simulink model "pmc_vlpr_s32k14x"  (Simulink 9.0)
settings: Solver=FixedStepDiscrete  StartTime=0.0  StopTime=10.0  FixedStep=0.001  RelTol=1e-3
InitFcn:
  | mbd_s32k_consistency_checks(bdroot(gcs));
undefined symbols (not defined in the file): LQFP
libraries: mbd_s32k1xx_ec_toolbox x14, simulink x1
Description:
  | This model demonstrates the "VLPR" functionality by setting the
  | processor to run in the Very low power run (VLPR) mode. When the SW3 button is
  | pressed, the processor runs into the VLPR mode. To exit the VLPR mode to RUN mode
  | SW2 button must be pressed.
  | 
  | Attention: The VLPR mode  disables most of the clocks. Using LPIT timer as interrupt
  | for the step function causes to halt processor when the VLPR mode is switched on. This
  | model uses VLPR timer (clocked by SIRC which is on in VLPR mode) as step function
  | trigger so the Step Tick Timer must be suppressed.
  | 
  | Validation: When the processor boots up, the RGB led lights up green and the processor
  | runs in the RUN mode. The RGB will toggle blue every half a second. When the SW3 is
  | pressed the processor enters the VLPR mode and the RGB turns red. The Blue light will
  | continue to toggle. When the SW2 is pressed the processor toggles the RGB led green and
  | the processor will run in RUN mode.
  | 
  | Optional: In order to measure the current consumption of the processor you can desolder
  | the R117 resistor (on the S32K144EVB board) and attach an ammeter on the J15 jumper.
  | 
  | Warning: Do NOT program the board while the uC is running in the low poer mode!
settings Model: Creator=NXP MBDT Team  LastModifiedBy=nxf35172
settings DataIOCC: ExternalInput=off  InitialState=off  SaveFormat=Dataset  SaveOutput=off  SignalLogging=off  SaveTime=off
settings OptimizationCC: DefaultParameterBehavior=Inlined  LifeSpan=1
settings DebuggingCC: UnderspecifiedInitializationDetection=Simplified  MergeDetectMultiDrivingBlocksExec=error  InheritedTsInSrcMsg=none  SingleTaskRateTransMsg=error  ParameterTunabilityLossMsg=error  UnconnectedInputMsg=error  UnconnectedOutputMsg=error  UnconnectedLineMsg=error  UnknownTsInhSupMsg=error  SFUnexpectedBacktrackingDiag=error  SFNoUnconditionalDefaultTransitionDiag=error
settings HardwareCC: ProdLargestAtomicInteger=Long  ProdLargestAtomicFloat=Double  ProdIntDivRoundTo=Zero  ProdEndianess=LittleEndian  ProdHWDeviceType=ARM Compatible->ARM Cortex
settings ModelReferenceCC: PropagateSignalLabelsOutOfModel=on
settings SFSimCC: SimBuildMode=sf_nonincremental_build  MATLABDynamicMemAlloc=off
settings RTWCC: SystemTargetFile=mbd_s32k.tlc  MakeCommand=mbd_s32k_make_rtw COPY_MDLREF_INCLUDES=0  TemplateMakefile=mbd_s32k.tmf  Description=Model Based Design Toolbox S32K14x Code Generation Target  GenerateReport=on  RetainRTWFile=on  IncludeHyperlinkInReport=on  LaunchReport=on  GenerateTraceInfo=on  GenerateTraceReport=on  GenerateTraceReportSl=on  GenerateTraceReportSf=on  GenerateTraceReportEml=on
settings CodeAppCC: ForceParamTrailComments=on  IgnoreCustomStorageClasses=off  OperatorAnnotations=on  SimulinkDataObjDesc=on  SFDataObjDesc=on  MATLABFcnDesc=on  InsertBlockDesc=on  MATLABSourceComments=on
settings STFCustomTargetCC: CombineOutputUpdateFcns=on  ERTCustomFileBanners=on  SupportContinuousTime=off  SupportNonInlinedSFcns=off  RemoveResetFunc=on  MATLABClassNameForMDSCustomization=Simulink.SoftwareTarget.ERTCustomization  GRTInterface=off  SystemTargetFile=mbd_s32k14.tlc
settings ERTTargetCC: MultiwordLength=2048  ParMdlRefBuildCompliant=off  CompOptLevelCompliant=off  ConcurrentExecutionCompliant=off  ModelStepFunctionPrototypeControlCompliant=off  CPPClassGenCompliant=off  UseToolchainInfoCompliant=off  InlinedParameterPlacement=NonHierarchical  ERTCustomFileTemplate=example_file_process.tlc  ConvertIfToSwitch=off  SuppressUnreachableDefaultCases=off
settings ConfigComp: CovMetricSettings=dwe  CovHtmlReporting=off  CovSaveCumulativeToWorkspaceVar=off  CovSaveSingleToWorkspaceVar=off  CovExternalEMLEnable=on

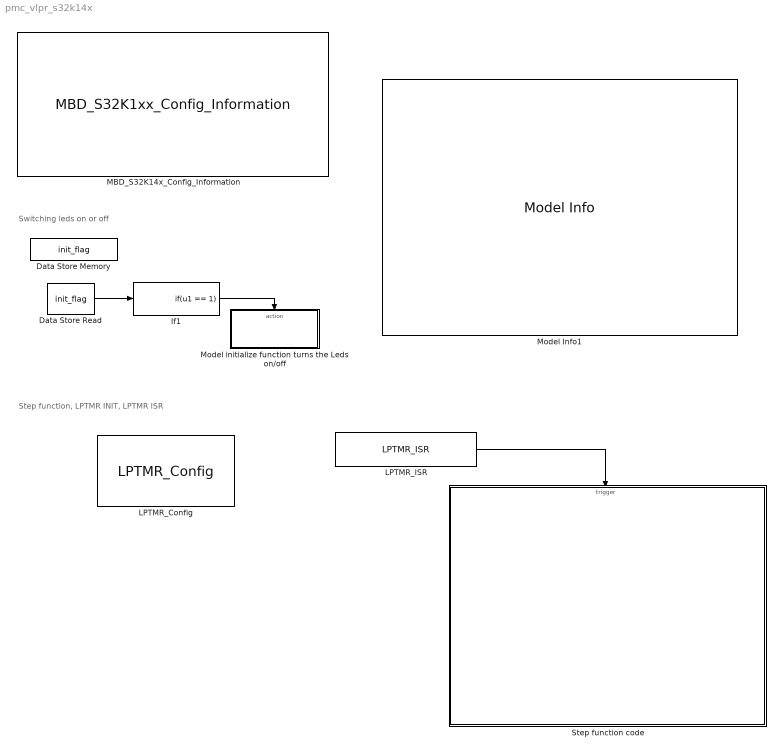
== system pmc_vlpr_s32k14x ==
  note: Switching leds on or off
  note: Step function, LPTMR INIT, LPTMR ISR
  Data Store Memory : DataStoreMemory  DataStoreName=init_flag  ReadBeforeWriteMsg=warning  WriteAfterWriteMsg=warning  WriteAfterReadMsg=warning  InitialValue=1  ShowAdditionalParam=off  OutDataTypeStr=boolean
  Data Store Read : DataStoreRead  DataStoreName=init_flag
  If1 : If  IfExpression=u1 == 1  ShowElse=off
  LPTMR_Config : mbd_s32k1xx_ec_toolbox/Core and System Blocks/LPTMR Blocks/LPTMR_Config  work_mode=Time Counter mode  compare_value=1000  compare_value_units=Microseconds  pin_select=Count pulses from pin alternative 1  pin_polarity=Count pulse on rising edge  pin_trgmux_source=Trigger function is disabled  pin_gpio=PTE11: [LPTMR0_ALT1 | Low Power Timer Input Channel]  show_adv_opts=on  input_clock=SIRC DIV2 clock  prescaler=Timer mode: prescaler 2, Glitch filter mode: invalid  bypass_prescaler=off  free_run=off  start_counter=on  enable_isr=on
  LPTMR_ISR : mbd_s32k1xx_ec_toolbox/Core and System Blocks/LPTMR Blocks/LPTMR_ISR
  MBD_S32K14x_Config_Information : mbd_s32k1xx_ec_toolbox/MBD_S32K1xx_Config_Information  mbdt_ver=0  disp_str=|  config_params=[]  mcu_target_name=S32K144  mcu_target_package=100-LQFP  mcu_target_sram_size=64KB  mcu_system_clock_freq=80  mcu_xtal_freq=External 8  mcu_steptick_timer=LPIT Channel 0  mcu_steptick_prio=15  ds_import_enable=on  target_compiler=GCC  target_memory=FLASH  gcc_target_compile_opts=-mcpu=cortex-m4 -mthumb -mfloat-abi=hard -mfpu=fpv4-sp-d16 -O1 -g -gstrict-dwarf  gcc_target_assemble_opts=-mcpu=cortex-m4 -mthumb -mfloat-abi=hard -mfpu=fpv4-sp-d16 -g  gcc_target_link_opts=-mcpu=cortex-m4 -mthumb -mfloat-abi=hard -mfpu=fpv4-sp-d16  gcc_target_default_lcf=on  gcc_target_user_lcf=S32K144_64_flash.ld  ghs_target_compile_opts=-cpu=cortexm4f -thumb -DARM_MATH_CM4 -fpu=vfpv4_d16 -fsingle -Ogeneral -Wundef -Wimplicit-int -Wshadow -Wtrigraphs --no_commons --gnu_asm -gnu99 -gdwarf-2 -G  ghs_target_assemble_opts=-cpu=cortexm4f -fpu=vfpv4_d16  ghs_target_link_opts=-cpu=cortexm4f -thumb -fpu=vfpv4_d16  ghs_target_default_lcf=on  ghs_target_user_lcf=S32K144_64_flash.ld  iar_target_compile_opts=--cpu=Cortex-M4F --thumb --fpu=VFPv4_sp -Ol -e --debug --dlib_config normal  iar_target_assemble_opts=--cpu Cortex-M4F --thumb --fpu VFPv4_sp  iar_target_link_opts=--no_exceptions --vfe --inline  iar_target_default_lcf=on  iar_target_user_lcf=S32K144_64_flash.icf  pil_download_enable=off  rbl_download_enable=on  rbl_start_delay=5000000  rbl_download_interface=OpenSDA  rbl_restart_request=off  rbl_com_port=Custom  rbl_com_port_custom=COM1  pil_download_rate=57600  pil_opensda_drive=Custom  pil_opensda_drive_custom=D  pil_uart_instance=0  pil_uart_rx=PTA2: [LPUART0_RX | Receive]  pil_uart_tx=PTA3: [LPUART0_TX | Transmit]  FTM_PWM_PcrCheckEnDis=on  FTM_Input_Edge_Inputs_PcrCheckEnDis=on  FTM_Dual_Edge_Inputs_PcrCheckEnDis=on  FTM_Quadrature_Inputs_PcrCheckEnDis=on  FTM_Hall_Sensor_Inputs_PcrCheckEnDis=on  LPTMR_PcrCheckEnDis=on  PIT_PcrCheckEnDis=on  RTC_PcrCheckEnDis=on  FlexCAN_PcrCheckEnDis=on  LIN_PcrCheckEnDis=on  FlexIO_PcrCheckEnDis=on  LPI2C_PcrCheckEnDis=on  LPSPI_PcrCheckEnDis=on  LPUART_PcrCheckEnDis=on  CMP_PcrCheckEnDis=on  GPIO_OutputPcrCheckEnDis=on  GPIO_InputPcrCheckEnDis=on  SBC_PcrCheckEnDis=on  AMMCLIB_PcrCheckEnDis=on  FM_PcrCheckEnDis=on  Profile_PcrCheckEnDis=on  ConfigParams_PcrCheckEnDis=on  ModelRef_PcrCheckEnDis=on  PDB0_PcrCheckEnDis=on  CSEc_PcrCheckEnDis=on  eDMA_PcrCheckEnDis=on  ADC_PcrCheckEnDis=on  WDOG_PcrCheckEnDis=on
      | Target : S32K144-64KB_SRAM
      | Package : 100-pin
      | System clock : 80 MHz
      | XTAL clock : External 8 MHz
      | Compiler : GCC
      | Target Type : FLASH
      | Download Code after build : (OpenSDA: D)
      | Step Tick Interrupt Priority : 10
  Model Info1 : simulink/Model-Wide Utilities/Model Info  Frame=off  DisplayStringWithTags=|  HorizontalTextAlignment=Left  LeftAlignmentValue=0.02
      | Model Name: %<ModelName>
      | 
      | Description: %<Description>
  Model initialize function turns the Leds on/off : Subsystem  TreatAsAtomicUnit=on
  Step function code : Subsystem
  wires:
  LPTMR_ISR/1 -> Step function code/Trigger
  Data Store Read/1 -> If1/1
  If1/1 -> Model initialize function turns the Leds on/off/Action

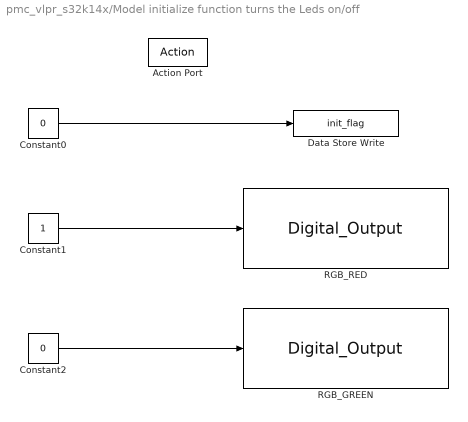
== system pmc_vlpr_s32k14x/Model initialize function turns the Leds on/off ==
  Action Port : ActionPort
  Constant0 : Constant  Value=0  OutDataTypeStr=boolean
  Constant1 : Constant  OutDataTypeStr=boolean
  Constant2 : Constant  Value=0  OutDataTypeStr=boolean
  Data Store Write : DataStoreWrite  DataStoreName=init_flag
  RGB_GREEN : mbd_s32k1xx_ec_toolbox/GPIO Blocks/Digital_Output  gpio_pin=PTD16: [PTD16 | Port D I/O]  init_val=Low  drive_strength=Low
  "RGB_RED " : mbd_s32k1xx_ec_toolbox/GPIO Blocks/Digital_Output  gpio_pin=PTD15: [PTD15 | Port D I/O]  init_val=Low  drive_strength=Low
  wires:
  Constant1/1 -> "RGB_RED "/1
  Constant0/1 -> Data Store Write/1
  Constant2/1 -> RGB_GREEN/1

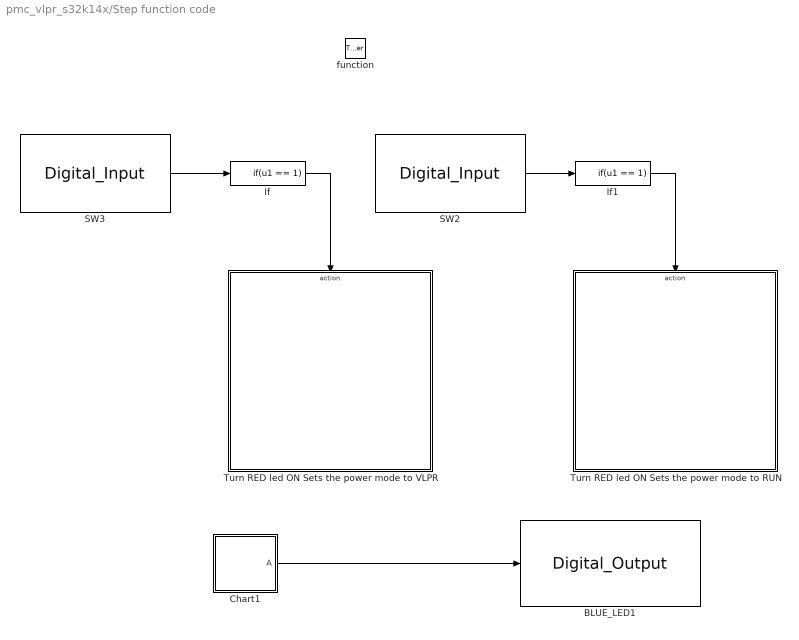
== system pmc_vlpr_s32k14x/Step function code ==
  function : TriggerPort  TriggerType=function-call  VariantControl=Variant
  BLUE_LED1 : mbd_s32k1xx_ec_toolbox/GPIO Blocks/Digital_Output  gpio_pin=PTD0: [PTD0 | Port D I/O]  init_val=Low  drive_strength=Low
  Chart1 : Stateflow chart  TreatAsAtomicUnit=on
  If : If  IfExpression=u1 == 1  ShowElse=off
  If1 : If  IfExpression=u1 == 1  ShowElse=off
  SW2 : mbd_s32k1xx_ec_toolbox/GPIO Blocks/Digital_Input  gpio_pin=PTC12: [PTC12 | Port C I/O]  pull_resistor=None  passive_filter=on
  SW3 : mbd_s32k1xx_ec_toolbox/GPIO Blocks/Digital_Input  gpio_pin=PTC13: [PTC13 | Port C I/O]  pull_resistor=None  passive_filter=on
  Turn RED led ON Sets the power mode to RUN : Subsystem  TreatAsAtomicUnit=on
  Turn RED led ON Sets the power mode to VLPR : Subsystem  TreatAsAtomicUnit=on
  wires:
  Chart1/1(" A") -> BLUE_LED1/1
  SW3/1 -> If/1
  If/1 -> Turn RED led ON Sets the power mode to VLPR/Action
  SW2/1 -> If1/1
  If1/1 -> Turn RED led ON Sets the power mode to RUN/Action

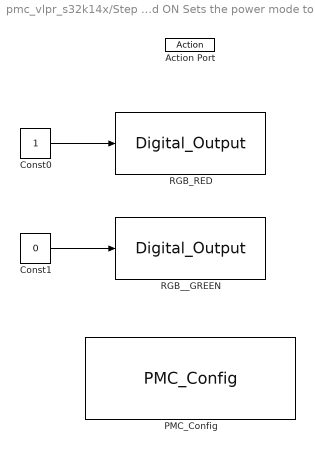
== system pmc_vlpr_s32k14x/Step function code/Turn RED led ON Sets the power mode to RUN ==
  Action Port : ActionPort
  Const0 : Constant  OutDataTypeStr=boolean
  Const1 : Constant  Value=0  OutDataTypeStr=boolean
  PMC_Config : mbd_s32k1xx_ec_toolbox/Core and System Blocks/PMC Blocks/PMC_Config  power_mode=Normal Operating (RUN)  sleep_on_exit=off  callback_before=off  callback_after=off  callback_before_after=off  show_adv_opts=off
  RGB_RED : mbd_s32k1xx_ec_toolbox/GPIO Blocks/Digital_Output  gpio_pin=PTD15: [PTD15 | Port D I/O]  init_val=Low  drive_strength=Low
  RGB__GREEN : mbd_s32k1xx_ec_toolbox/GPIO Blocks/Digital_Output  gpio_pin=PTD16: [PTD16 | Port D I/O]  init_val=Low  drive_strength=Low
  wires:
  Const0/1 -> RGB_RED/1
  Const1/1 -> RGB__GREEN/1

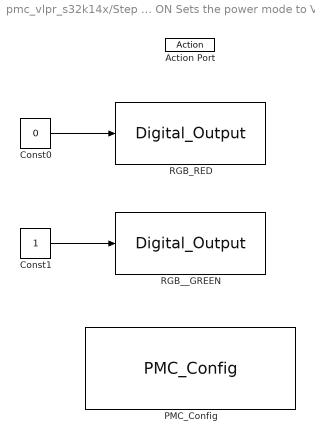
== system pmc_vlpr_s32k14x/Step function code/Turn RED led ON Sets the power mode to VLPR ==
  Action Port : ActionPort
  Const0 : Constant  Value=0  OutDataTypeStr=boolean
  Const1 : Constant  OutDataTypeStr=boolean
  PMC_Config : mbd_s32k1xx_ec_toolbox/Core and System Blocks/PMC Blocks/PMC_Config  power_mode=Very Low Power Run (VLPR)  sleep_on_exit=off  callback_before=off  callback_after=off  callback_before_after=off  show_adv_opts=off
  RGB_RED : mbd_s32k1xx_ec_toolbox/GPIO Blocks/Digital_Output  gpio_pin=PTD15: [PTD15 | Port D I/O]  init_val=Low  drive_strength=Low
  RGB__GREEN : mbd_s32k1xx_ec_toolbox/GPIO Blocks/Digital_Output  gpio_pin=PTD16: [PTD16 | Port D I/O]  init_val=Low  drive_strength=Low
  wires:
  Const0/1 -> RGB_RED/1
  Const1/1 -> RGB__GREEN/1

== stateflow chart Step function code/Chart1 ==
  state A
    entry: cnt = cnt +1;
  state A1
    entry: cnt = cnt - 1;
  (default) -> A : {cnt = 0}
  A -> A [order 2]
  A -> A1 [order 1] : [cnt == 500]
  A1 -> A [order 1] : [cnt  == 0]
  A1 -> A1 [order 2]
  data: A output boolean [0..1]; cnt local double
